simulink model "practica8_simulink_"  (R2024b)
settings: Solver=VariableStepAuto  StartTime=0.0  StopTime=10.0  RelTol=1e-3
values from neighbouring files (symbols this model uses):
  b = 0.0012    [practica_8_ODE.m]    (also in valores.m)
  J = 0.001    [practica_8_ODE.m]    (also in valores.m)
  ke = 0.01    [practica_8_ODE.m]    (also in valores.m)
  Kt = 0.01    [practica_8_ODE.m]    (also in valores.m)
  La = 0.023    [practica_8_ODE.m]    (also in valores.m)
  R = 2    [practica_8_ODE.m]    (also in valores.m)
  Va = 5    [practica_8_ODE.m]    (also in valores.m)

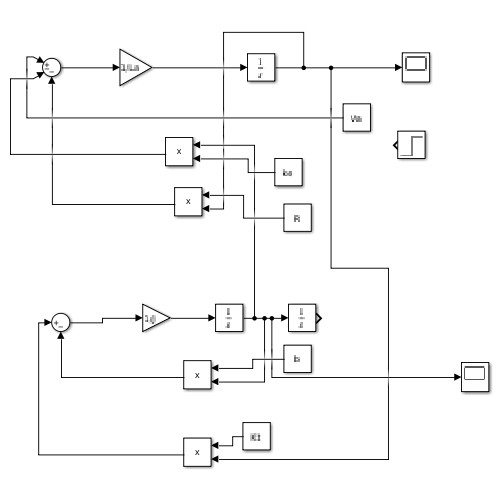
[thumbnail: Simulink's stored preview of the top-level diagram]
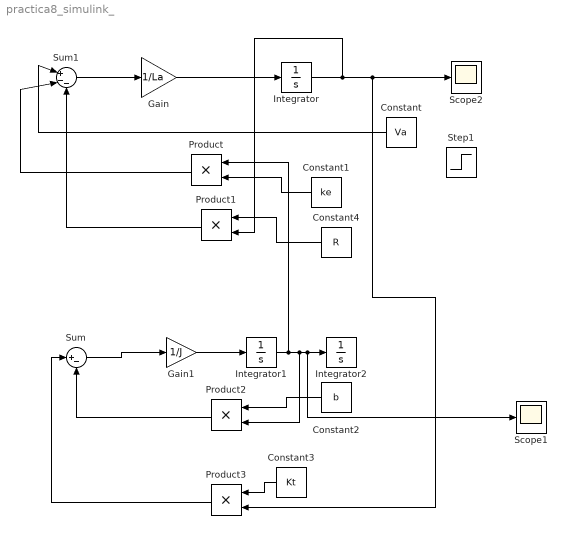
== system practica8_simulink_ ==
  Constant : Constant  Value=Va
  Constant1 : Constant  Value=ke
  Constant2 : Constant  Value=b
  Constant3 : Constant  Value=Kt
  Constant4 : Constant  Value=R
  Gain : Gain  Gain=1/La
  Gain1 : Gain  Gain=1/J
  Integrator : Integrator
  Integrator1 : Integrator
  Integrator2 : Integrator
  Product{,1..3} (4 alike) : Product
  Scope1 : Scope
  Scope2 : Scope
  Step1 : Step  Time=0  After=5  SampleTime=0
  Sum : Sum  Inputs=|+-
  Sum1 : Sum  Inputs=|+--
  wires:
  Sum1/1 -> Gain/1
  Constant/1 -> Sum1/1
  Constant1/1 -> Product/2
  Product/1 -> Sum1/2
  Constant4/1 -> Product1/1
  Sum/1 -> Gain1/1
  Gain1/1 -> Integrator1/1
  Product1/1 -> Sum1/3
  Constant2/1 -> Product2/1
  Constant3/1 -> Product3/1
  Product2/1 -> Sum/2
  Product3/1 -> Sum/1
  Integrator1/1 -> Product/1, Product2/2, Scope1/1, Integrator2/1
  Gain/1 -> Integrator/1
  Integrator/1 -> Product1/2, Scope2/1, Product3/2
